simulink model "mrefrobotarm_modified_previous_y_previous_u_previous_ref_Thao"  (R2018b)
settings: Solver=FixedStepAuto  StartTime=0.0  StopTime=10  RelTol=1e-3  AbsTol=1e-6
undefined symbols (not defined in the file or in its folder): sfunxy2
libraries: neural x668, simulink x1
(part 16 of 21)

== system mrefrobotarm_modified_previous_y_previous_u_previous_ref_Thao/trimmed_2_report/Layer 2/Delays 1 ==
  "p{2}" : Inport  PortDimensions=50
      mask Display: e = 0.06;c1 = [120 230 180]/255;c2 = ([120 230 180]+0)/(256+128);c3 = ([120 230 180]+128)/(256+128);patch([0 1 1 0],[0 0 1 1],c1);patch([0 1 1 1-e 1-e 0+e],[0 0 1 1-e 0+e 0+e],c2);patch([0 0 1 1-e 0+e 0+e],[0 1 1 1-e 1-e 0+e],c3);plot([0 1 1 0 0],[0 0 1 1 0]);
  mux : Mux  Inputs=1
      mask Display: e = 0.06;c1 = [120 150 230]/255;c2 = ([120 150 230]+0)/383;c3 = ([120 150 230]+128)/383;patch([0 1 1 0],[0 0 1 1],c1);patch([0 1 1 1-e 1-e 0+e],[0 0 1 1-e 0+e 0+e],c2);patch([0 0 1 1-e 0+e 0+e],[0 1 1 1-e 1-e 0+e],c3);plot([0 1 1 0 0],[0 0 1 1 0]);disp('Mux')
  "pd{2,1}" : Outport
      mask Display: e = 0.06;c1 = [120 230 180]/255;c2 = ([120 230 180]+0)/(256+128);c3 = ([120 230 180]+128)/(256+128);patch([0 1 1 0],[0 0 1 1],c1);patch([0 1 1 1-e 1-e 0+e],[0 0 1 1-e 0+e 0+e],c2);patch([0 0 1 1-e 0+e 0+e],[0 1 1 1-e 1-e 0+e],c3);plot([0 1 1 0 0],[0 0 1 1 0]);
  wires:
  "p{2}"/1 -> mux/1
  mux/1 -> "pd{2,1}"/1

== system mrefrobotarm_modified_previous_y_previous_u_previous_ref_Thao/trimmed_2_report/Layer 2/LW{2,1} ==
  "ad{2,1}" : Inport  PortDimensions=50
      mask Display: e = 0.06;c1 = [120 230 180]/255;c2 = ([120 230 180]+0)/(256+128);c3 = ([120 230 180]+128)/(256+128);patch([0 1 1 0],[0 0 1 1],c1);patch([0 1 1 1-e 1-e 0+e],[0 0 1 1-e 0+e 0+e],c2);patch([0 0 1 1-e 0+e 0+e],[0 1 1 1-e 1-e 0+e],c3);plot([0 1 1 0 0],[0 0 1 1 0]);
  "IW{2,1}(1,:)'" : Constant  Value=[-0.534499281996474007172537312726490199565887451171875;0.050521392035346612825463807894266210496425628662109375;-0.1237457148938286011219389592952211387455463409423828125;0.27380803107087559045140778835047967731952667236328125;-0.158040380072445307835238281768397428095340728759765625;0.0117056595849677480547512686825939454138278961181640625;0.0221259878671266306537912527119260630570352077484130859375;-0.021458436433733317494354508880860521458089351654052734375;0.51989139454196420242482190587907098233699798583984375;0.227624128585074136932320243431604467332363128662109375;0.01291812527474923803783024567337633925490081310272216796875;0.394990958343573284050620486596017144620418548583984375;-0.31659097344442466148706216699793003499507904052734375;0.056111623746644932742011491200173622928559780120849609375;0.0645209389209373818108161913187359459698200225830078125;-0.026299150809179223931000279890213278122246265411376953125;-0.21062033219300591024847335575032047927379608154296875;0.4157878309067550848254768425249494612216949462890625;-0.1393911657788584890216299072562833316624164581298828125;0.007629605525119244335829904457568773068487644195556640625;-0.10964960705708633181831856973076355643570423126220703125;0.0231723744225558851705937257747791591100394725799560546875;-0.0049260595140393458046812469319775118492543697357177734375;-0.1840150338819656339328645344721735455095767974853515625;-0.102919672671898665416989615550846792757511138916015625;-0.00142893900606726360902332118030244600959122180938720703125;0.4164215191432472096266792505048215389251708984375;0.047497327884583662171991136347060091793537139892578125;-0.3258562173255992178155793226324021816253662109375;0.07218624218910708878471638172413804568350315093994140625;-0.000558610505585981249876414977961758268065750598907470703125;0.0227008210951530169097178912807066808454692363739013671875;0.004049470967297652025662646479986506165005266666412353515625;0.3794867924264113678844978494453243911266326904296875;-0.08706497710380935173279937089318991638720035552978515625;-0.299736725995607578010293536863173358142375946044921875;-0.046645176662323352412276022960213595069944858551025390625;0.2332394792535505689823338570931809954345226287841796875;0.0599754359488125776689315671319491229951381683349609375;0.158592158288105355978814259287901222705841064453125;0.061120750010903390769811949212453328073024749755859375;0.28961701664959627056106228337739594280719757080078125;0.057366268033513988233718094988944358192384243011474609375;0.05267609339257973977144189348109648562967777252197265625;0.0773590555953053982118916565013932995498180389404296875;-0.0394302645710693788760892175560002215206623077392578125;0.0381727970716883024948629099526442587375640869140625;-0.32777144511634259682608671937487088143825531005859375;0.329085099439463346637779750381014309823513031005859375;0.0716558723123885410455358169201645068824291229248046875]
      mask Display: e = 0.06;c1 = [120 150 230]/255;c2 = ([120 150 230]+0)/383;c3 = ([120 150 230]+128)/383;patch([0 1 1 0],[0 0 1 1],c1);patch([0 1 1 1-e 1-e 0+e],[0 0 1 1-e 0+e 0+e],c2);patch([0 0 1 1-e 0+e 0+e],[0 1 1 1-e 1-e 0+e],c3);plot([0 1 1 0 0],[0 0 1 1 0]);disp('weights');
  Mux : Mux  Inputs=1
      mask Display: e = 0.06;c1 = [120 150 230]/255;c2 = ([120 150 230]+0)/383;c3 = ([120 150 230]+128)/383;patch([0 1 1 0],[0 0 1 1],c1);patch([0 1 1 1-e 1-e 0+e],[0 0 1 1-e 0+e 0+e],c2);patch([0 0 1 1-e 0+e 0+e],[0 1 1 1-e 1-e 0+e],c3);plot([0 1 1 0 0],[0 0 1 1 0]);disp('Mux');
  dotprod1 : neural/Weight Functions/dotprod
  "lz{2,1}" : Outport
      mask Display: e = 0.06;c1 = [120 230 180]/255;c2 = ([120 230 180]+0)/(256+128);c3 = ([120 230 180]+128)/(256+128);patch([0 1 1 0],[0 0 1 1],c1);patch([0 1 1 1-e 1-e 0+e],[0 0 1 1-e 0+e 0+e],c2);patch([0 0 1 1-e 0+e 0+e],[0 1 1 1-e 1-e 0+e],c3);plot([0 1 1 0 0],[0 0 1 1 0]);
  wires:
  "IW{2,1}(1,:)'"/1 -> dotprod1/1
  "ad{2,1}"/1 -> dotprod1/2
  dotprod1/1 -> Mux/1
  Mux/1 -> "lz{2,1}"/1

== system mrefrobotarm_modified_previous_y_previous_u_previous_ref_Thao/trimmed_cex/Layer 1/Delays 1 ==
  "p{1}" : Inport  PortDimensions=10
      mask Display: e = 0.06;c1 = [120 230 180]/255;c2 = ([120 230 180]+0)/(256+128);c3 = ([120 230 180]+128)/(256+128);patch([0 1 1 0],[0 0 1 1],c1);patch([0 1 1 1-e 1-e 0+e],[0 0 1 1-e 0+e 0+e],c2);patch([0 0 1 1-e 0+e 0+e],[0 1 1 1-e 1-e 0+e],c3);plot([0 1 1 0 0],[0 0 1 1 0]);
  mux : Mux  Inputs=1
      mask Display: e = 0.06;c1 = [120 150 230]/255;c2 = ([120 150 230]+0)/383;c3 = ([120 150 230]+128)/383;patch([0 1 1 0],[0 0 1 1],c1);patch([0 1 1 1-e 1-e 0+e],[0 0 1 1-e 0+e 0+e],c2);patch([0 0 1 1-e 0+e 0+e],[0 1 1 1-e 1-e 0+e],c3);plot([0 1 1 0 0],[0 0 1 1 0]);disp('Mux')
  "pd{1,1}" : Outport
      mask Display: e = 0.06;c1 = [120 230 180]/255;c2 = ([120 230 180]+0)/(256+128);c3 = ([120 230 180]+128)/(256+128);patch([0 1 1 0],[0 0 1 1],c1);patch([0 1 1 1-e 1-e 0+e],[0 0 1 1-e 0+e 0+e],c2);patch([0 0 1 1-e 0+e 0+e],[0 1 1 1-e 1-e 0+e],c3);plot([0 1 1 0 0],[0 0 1 1 0]);
  wires:
  "p{1}"/1 -> mux/1
  mux/1 -> "pd{1,1}"/1

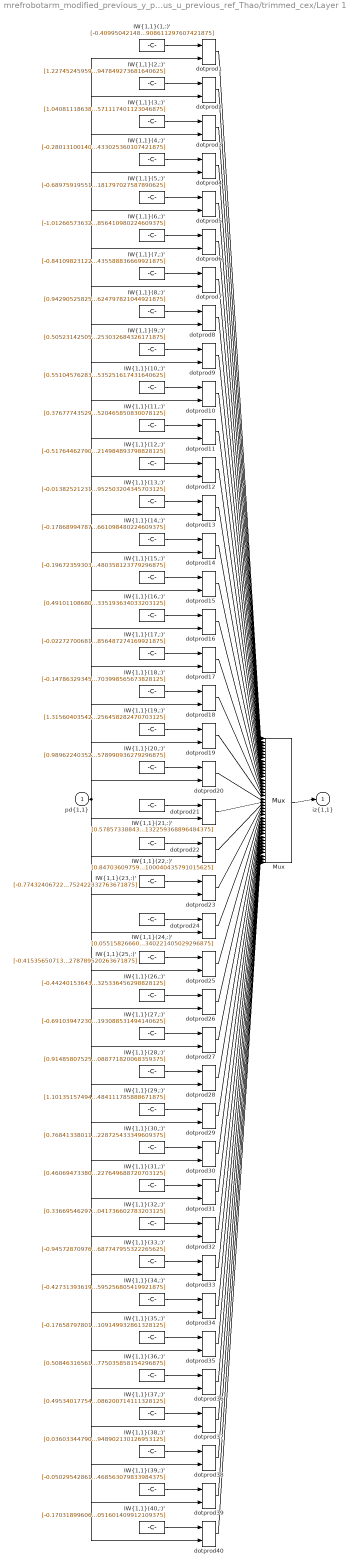
== system mrefrobotarm_modified_previous_y_previous_u_previous_ref_Thao/trimmed_cex/Layer 1/IW{1,1} ==
  "pd{1,1}" : Inport  PortDimensions=10
      mask Display: e = 0.06;c1 = [120 230 180]/255;c2 = ([120 230 180]+0)/(256+128);c3 = ([120 230 180]+128)/(256+128);patch([0 1 1 0],[0 0 1 1],c1);patch([0 1 1 1-e 1-e 0+e],[0 0 1 1-e 0+e 0+e],c2);patch([0 0 1 1-e 0+e 0+e],[0 1 1 1-e 1-e 0+e],c3);plot([0 1 1 0 0],[0 0 1 1 0]);
  "IW{1,1}(1,:)'" : Constant  Value=[-0.409950421486075355925748908703099004924297332763671875;-0.2664484226456824700335346278734505176544189453125;0.82215987443999594130872310415725223720073699951171875;-0.8070804278638721296346147937583737075328826904296875;-0.6354261914999630445066713946289382874965667724609375;0.93223383088760336523392879826133139431476593017578125;-0.478382274522026751384373710607178509235382080078125;-0.64553475014590000480296794194146059453487396240234375;0.60487535966275285392867999689769931137561798095703125;-0.154506010113978298203818440015311352908611297607421875]
      mask Display: e = 0.06;c1 = [120 150 230]/255;c2 = ([120 150 230]+0)/383;c3 = ([120 150 230]+128)/383;patch([0 1 1 0],[0 0 1 1],c1);patch([0 1 1 1-e 1-e 0+e],[0 0 1 1-e 0+e 0+e],c2);patch([0 0 1 1-e 0+e 0+e],[0 1 1 1-e 1-e 0+e],c3);plot([0 1 1 0 0],[0 0 1 1 0]);disp('Weights');
  "IW{1,1}(10,:)'" : Constant  Value=[0.55104576283990980289928529600729234516620635986328125;0.70635327144264181686850179175962693989276885986328125;1.0688781204485005016380227971239946782588958740234375;0.2351630117278747655884529876857413910329341888427734375;0.18201702354305349107477240977459587156772613525390625;-0.55143005136851630521022116226959042251110076904296875;-0.86246809425289316930474114997196011245250701904296875;-0.9777826678231626988946345591102726757526397705078125;0.74981547833765638255698604552890174090862274169921875;0.55583250060019795402155295960255898535251617431640625]
      mask Display: e = 0.06;c1 = [120 150 230]/255;c2 = ([120 150 230]+0)/383;c3 = ([120 150 230]+128)/383;patch([0 1 1 0],[0 0 1 1],c1);patch([0 1 1 1-e 1-e 0+e],[0 0 1 1-e 0+e 0+e],c2);patch([0 0 1 1-e 0+e 0+e],[0 1 1 1-e 1-e 0+e],c3);plot([0 1 1 0 0],[0 0 1 1 0]);disp('Weights');
  "IW{1,1}(11,:)'" : Constant  Value=[0.3767774352905917112366296350955963134765625;0.2009752253063678828493010541933472268283367156982421875;-0.89354895099178488493407712667249143123626708984375;0.6899875287137533508285969219286926090717315673828125;1.125933724805846747329951540450565516948699951171875;0.54802615696479095586113317040144465863704681396484375;0.38602265314686545760736180454841814935207366943359375;-0.31980146358828631658610675003728829324245452880859375;-1.0052964528057055648702089456492103636264801025390625;0.327354157170351378614014947743271477520465850830078125]
      mask Display: e = 0.06;c1 = [120 150 230]/255;c2 = ([120 150 230]+0)/383;c3 = ([120 150 230]+128)/383;patch([0 1 1 0],[0 0 1 1],c1);patch([0 1 1 1-e 1-e 0+e],[0 0 1 1-e 0+e 0+e],c2);patch([0 0 1 1-e 0+e 0+e],[0 1 1 1-e 1-e 0+e],c3);plot([0 1 1 0 0],[0 0 1 1 0]);disp('Weights');
  "IW{1,1}(12,:)'" : Constant  Value=[-0.5176446279089115254379294128739275038242340087890625;0.74329648028114936320065453401184640824794769287109375;0.56129611953699132254058667967910878360271453857421875;0.6656237941179730110974333001649938523769378662109375;0.17927298805446090224080535335815511643886566162109375;1.010790447986693152415682561695575714111328125;0.8347516775559349344604243015055544674396514892578125;-0.2256657861482148919041179624400683678686618804931640625;0.2438529279834821539285627522986033000051975250244140625;0.79710465235954064411316721816547214984893798828125]
      mask Display: e = 0.06;c1 = [120 150 230]/255;c2 = ([120 150 230]+0)/383;c3 = ([120 150 230]+128)/383;patch([0 1 1 0],[0 0 1 1],c1);patch([0 1 1 1-e 1-e 0+e],[0 0 1 1-e 0+e 0+e],c2);patch([0 0 1 1-e 0+e 0+e],[0 1 1 1-e 1-e 0+e],c3);plot([0 1 1 0 0],[0 0 1 1 0]);disp('Weights');
  "IW{1,1}(13,:)'" : Constant  Value=[-0.0138252123130195199440795050804808852262794971466064453125;0.7310768485028218410803901861072517931461334228515625;0.1793313597198371578400610815151594579219818115234375;0.03382004408312382082169023078677128069102764129638671875;-1.7686173826988913493352129080449230968952178955078125;-0.25051326753296521143710151591221801936626434326171875;1.213436044436186467265770261292345821857452392578125;0.26416181179519904187458223532303236424922943115234375;-0.2117864442757750598200772174095618538558483123779296875;-0.43316444584072766321725111993146128952503204345703125]
      mask Display: e = 0.06;c1 = [120 150 230]/255;c2 = ([120 150 230]+0)/383;c3 = ([120 150 230]+128)/383;patch([0 1 1 0],[0 0 1 1],c1);patch([0 1 1 1-e 1-e 0+e],[0 0 1 1-e 0+e 0+e],c2);patch([0 0 1 1-e 0+e 0+e],[0 1 1 1-e 1-e 0+e],c3);plot([0 1 1 0 0],[0 0 1 1 0]);disp('Weights');
  "IW{1,1}(14,:)'" : Constant  Value=[-0.178689947872833265751779663332854397594928741455078125;-0.6214830678008553821456416699220426380634307861328125;0.301565599171200349193355805255123414099216461181640625;0.282215738197436449841148942141444422304630279541015625;-1.235070373536440779815848145517520606517791748046875;0.0018266847157617609187507667911631870083510875701904296875;0.0304094742715033151958525792224463657476007938385009765625;0.9682731964107362809812684645294211804866790771484375;0.63588548799484378992730171376024372875690460205078125;0.79038843670227298954245043205446563661098480224609375]
      mask Display: e = 0.06;c1 = [120 150 230]/255;c2 = ([120 150 230]+0)/383;c3 = ([120 150 230]+128)/383;patch([0 1 1 0],[0 0 1 1],c1);patch([0 1 1 1-e 1-e 0+e],[0 0 1 1-e 0+e 0+e],c2);patch([0 0 1 1-e 0+e 0+e],[0 1 1 1-e 1-e 0+e],c3);plot([0 1 1 0 0],[0 0 1 1 0]);disp('Weights');
  "IW{1,1}(15,:)'" : Constant  Value=[-0.1967235930329597481946990455980994738638401031494140625;0.4999398005660731225674453526153229176998138427734375;0.89412234324233430537987032948876731097698211669921875;0.05945266912088405242275968021203880198299884796142578125;0.0474482273376281848964453047301503829658031463623046875;0.3036461092060902533518174095661379396915435791015625;-0.15896471182623905793462881774757988750934600830078125;-0.9253496196720145672287571869674138724803924560546875;0.918719060230821948920265640481375157833099365234375;-0.900185313959386501636572575080208480358123779296875]
      mask Display: e = 0.06;c1 = [120 150 230]/255;c2 = ([120 150 230]+0)/383;c3 = ([120 150 230]+128)/383;patch([0 1 1 0],[0 0 1 1],c1);patch([0 1 1 1-e 1-e 0+e],[0 0 1 1-e 0+e 0+e],c2);patch([0 0 1 1-e 0+e 0+e],[0 1 1 1-e 1-e 0+e],c3);plot([0 1 1 0 0],[0 0 1 1 0]);disp('Weights');
  "IW{1,1}(16,:)'" : Constant  Value=[0.491011086807734031811634167752345092594623565673828125;0.155186933005624305703662457744940184056758880615234375;-0.11711099155229769130937000909398193471133708953857421875;-0.66276689623297635467480404258822090923786163330078125;-0.5422964498312499159737853915430605411529541015625;0.304146121397555424525904754773364402353763580322265625;0.887358139122755407157683293917216360569000244140625;-0.99099461583372683293191585107706487178802490234375;0.3830059630076496635098237675265409052371978759765625;0.27587055069574983878766261113923974335193634033203125]
      mask Display: e = 0.06;c1 = [120 150 230]/255;c2 = ([120 150 230]+0)/383;c3 = ([120 150 230]+128)/383;patch([0 1 1 0],[0 0 1 1],c1);patch([0 1 1 1-e 1-e 0+e],[0 0 1 1-e 0+e 0+e],c2);patch([0 0 1 1-e 0+e 0+e],[0 1 1 1-e 1-e 0+e],c3);plot([0 1 1 0 0],[0 0 1 1 0]);disp('Weights');
  "IW{1,1}(17,:)'" : Constant  Value=[-0.0227270068157796149843630217901591095142066478729248046875;-0.0033446203266591680025587862701286212541162967681884765625;0.555597040712585421573521671234630048274993896484375;0.4055619247689070672180378096527419984340667724609375;-0.69873436239766750777135939642903394997119903564453125;-0.69174437201428318200413514205138199031352996826171875;-0.14958891890921821588023021831759251654148101806640625;1.146594252841719008273457802715711295604705810546875;1.0912485097967479230618437213706783950328826904296875;0.69285833323481404999455435245181433856487274169921875]
      mask Display: e = 0.06;c1 = [120 150 230]/255;c2 = ([120 150 230]+0)/383;c3 = ([120 150 230]+128)/383;patch([0 1 1 0],[0 0 1 1],c1);patch([0 1 1 1-e 1-e 0+e],[0 0 1 1-e 0+e 0+e],c2);patch([0 0 1 1-e 0+e 0+e],[0 1 1 1-e 1-e 0+e],c3);plot([0 1 1 0 0],[0 0 1 1 0]);disp('Weights');
  "IW{1,1}(18,:)'" : Constant  Value=[-0.1478632934526930842178416014576214365661144256591796875;-0.3452155889878729677633373285061679780483245849609375;-0.0966016042904927763057543188551790080964565277099609375;-0.56056969383534227535648142293212004005908966064453125;-1.499417823985652820084624181617982685565948486328125;0.89052501293365116108446954967803321778774261474609375;-0.5465292024094947631596141945919953286647796630859375;0.54948094360087551546456552387098781764507293701171875;0.08803384133689766410935106932811322622001171112060546875;0.561317847656468860151335320551879703998565673828125]
      mask Display: e = 0.06;c1 = [120 150 230]/255;c2 = ([120 150 230]+0)/383;c3 = ([120 150 230]+128)/383;patch([0 1 1 0],[0 0 1 1],c1);patch([0 1 1 1-e 1-e 0+e],[0 0 1 1-e 0+e 0+e],c2);patch([0 0 1 1-e 0+e 0+e],[0 1 1 1-e 1-e 0+e],c3);plot([0 1 1 0 0],[0 0 1 1 0]);disp('Weights');
  "IW{1,1}(19,:)'" : Constant  Value=[1.31560403542571524582172060036100447177886962890625;0.8777692427769456795516589409089647233486175537109375;-0.205947039131328335503923199212295003235340118408203125;0.498609152543595890438865581018035300076007843017578125;-0.01839913800753746608851457722266786731779575347900390625;-0.498700799665831306928254207377904094755649566650390625;-0.42702038547360976483702188488678075373172760009765625;0.98979145575477545104803311915020458400249481201171875;0.096199212682389123596493618606473319232463836669921875;-0.2748632724632014134868995824945159256458282470703125]
      mask Display: e = 0.06;c1 = [120 150 230]/255;c2 = ([120 150 230]+0)/383;c3 = ([120 150 230]+128)/383;patch([0 1 1 0],[0 0 1 1],c1);patch([0 1 1 1-e 1-e 0+e],[0 0 1 1-e 0+e 0+e],c2);patch([0 0 1 1-e 0+e 0+e],[0 1 1 1-e 1-e 0+e],c3);plot([0 1 1 0 0],[0 0 1 1 0]);disp('Weights');
  "IW{1,1}(2,:)'" : Constant  Value=[1.2274524595998828058185381451039575040340423583984375;-0.1858982387281616077689960775387589819729328155517578125;0.028275394747831437969320944603168754838407039642333984375;0.0847112914180939979846840515165240503847599029541015625;-1.1893226383913002575098971647094003856182098388671875;-0.06498424728492711854865859777419245801866054534912109375;1.1521911516761191851543344455421902239322662353515625;-0.285463137559759216888011224000365473330020904541015625;-1.181173392303688896021185428253374993801116943359375;-0.6258040532702013880594904549070633947849273681640625]
      mask Display: e = 0.06;c1 = [120 150 230]/255;c2 = ([120 150 230]+0)/383;c3 = ([120 150 230]+128)/383;patch([0 1 1 0],[0 0 1 1],c1);patch([0 1 1 1-e 1-e 0+e],[0 0 1 1-e 0+e 0+e],c2);patch([0 0 1 1-e 0+e 0+e],[0 1 1 1-e 1-e 0+e],c3);plot([0 1 1 0 0],[0 0 1 1 0]);disp('Weights');
  "IW{1,1}(20,:)'" : Constant  Value=[0.9896224035276339758837593763018958270549774169921875;-0.44305668527520125632435110674123279750347137451171875;0.70981606561427990076396099539124406874179840087890625;-1.1297168139596982516792422757134772837162017822265625;0.848697028814358045423205112456344068050384521484375;0.4557425970205557508307947500725276768207550048828125;-0.39557951689199721823086974836769513785839080810546875;-0.00146782704480703796168228336682659573853015899658203125;0.2214522806691265888190400801249779760837554931640625;-0.132984556624309024908114906793343834578990936279296875]
      mask Display: e = 0.06;c1 = [120 150 230]/255;c2 = ([120 150 230]+0)/383;c3 = ([120 150 230]+128)/383;patch([0 1 1 0],[0 0 1 1],c1);patch([0 1 1 1-e 1-e 0+e],[0 0 1 1-e 0+e 0+e],c2);patch([0 0 1 1-e 0+e 0+e],[0 1 1 1-e 1-e 0+e],c3);plot([0 1 1 0 0],[0 0 1 1 0]);disp('Weights');
  "IW{1,1}(21,:)'" : Constant  Value=[0.57857338843473637979286650079302489757537841796875;0.55341504998858115360604870147653855383396148681640625;-0.64653962666199527031807292587473057210445404052734375;-0.5862476181018936305378019824274815618991851806640625;-0.35438450623822148610742033270071260631084442138671875;0.510302004487602101079346539336256682872772216796875;-0.9929389094367564450038798895548097789287567138671875;-0.74814260248213215742651982509414665400981903076171875;-0.90267234096774806584306816148455254733562469482421875;0.423604583182045801859061384675442241132259368896484375]
      mask Display: e = 0.06;c1 = [120 150 230]/255;c2 = ([120 150 230]+0)/383;c3 = ([120 150 230]+128)/383;patch([0 1 1 0],[0 0 1 1],c1);patch([0 1 1 1-e 1-e 0+e],[0 0 1 1-e 0+e 0+e],c2);patch([0 0 1 1-e 0+e 0+e],[0 1 1 1-e 1-e 0+e],c3);plot([0 1 1 0 0],[0 0 1 1 0]);disp('Weights');
  "IW{1,1}(22,:)'" : Constant  Value=[0.84703609759596532047254413555492646992206573486328125;-0.7880910829087459656960845677531324326992034912109375;-0.6116141806369055355929731376818381249904632568359375;-0.72231053399220801480851150699891149997711181640625;-0.6838583880533806169665922425338067114353179931640625;0.45809248458162443728980406376649625599384307861328125;-0.46923654407256443210627594453399069607257843017578125;-0.489852123921882542934014281854615546762943267822265625;-0.84453888161475798579402862742426805198192596435546875;0.2119728726749436076293164887829334475100040435791015625]
      mask Display: e = 0.06;c1 = [120 150 230]/255;c2 = ([120 150 230]+0)/383;c3 = ([120 150 230]+128)/383;patch([0 1 1 0],[0 0 1 1],c1);patch([0 1 1 1-e 1-e 0+e],[0 0 1 1-e 0+e 0+e],c2);patch([0 0 1 1-e 0+e 0+e],[0 1 1 1-e 1-e 0+e],c3);plot([0 1 1 0 0],[0 0 1 1 0]);disp('Weights');
  "IW{1,1}(23,:)'" : Constant  Value=[-0.77432406722360103135116560224560089409351348876953125;0.2209649232498732962515219924171105958521366119384765625;0.46444341998348026567811075437930412590503692626953125;-0.6595292492139612772206191948498599231243133544921875;0.134455139336463080912409395750728435814380645751953125;-1.10985874298612419153187147458083927631378173828125;-1.12233395519971512754864306771196424961090087890625;1.1289026833873487820625314270728267729282379150390625;0.49296594290608830579714094710652716457843780517578125;-0.1470205149079321926830488109771977178752422332763671875]
      mask Display: e = 0.06;c1 = [120 150 230]/255;c2 = ([120 150 230]+0)/383;c3 = ([120 150 230]+128)/383;patch([0 1 1 0],[0 0 1 1],c1);patch([0 1 1 1-e 1-e 0+e],[0 0 1 1-e 0+e 0+e],c2);patch([0 0 1 1-e 0+e 0+e],[0 1 1 1-e 1-e 0+e],c3);plot([0 1 1 0 0],[0 0 1 1 0]);disp('Weights');
  "IW{1,1}(24,:)'" : Constant  Value=[0.0551582666045678238209148958048899658024311065673828125;-0.2255705806114211287027870866950252093374729156494140625;-0.1126119364538074318904392612239462323486804962158203125;-0.7413220356632257423967757858918048441410064697265625;0.54959437813839329134424360745470039546489715576171875;0.94089820560549319861110006968374364078044891357421875;-0.2087613420724725721289161128879641182720661163330078125;-0.0106507648017074955937300018149471725337207317352294921875;1.180621398067102756357371617923490703105926513671875;-0.9673907138311139686237538626301102340221405029296875]
      mask Display: e = 0.06;c1 = [120 150 230]/255;c2 = ([120 150 230]+0)/383;c3 = ([120 150 230]+128)/383;patch([0 1 1 0],[0 0 1 1],c1);patch([0 1 1 1-e 1-e 0+e],[0 0 1 1-e 0+e 0+e],c2);patch([0 0 1 1-e 0+e 0+e],[0 1 1 1-e 1-e 0+e],c3);plot([0 1 1 0 0],[0 0 1 1 0]);disp('Weights');
  "IW{1,1}(25,:)'" : Constant  Value=[-0.415356507133745889159825992464902810752391815185546875;0.86324940583818221551126725898939184844493865966796875;0.99650446455441699100674668443389236927032470703125;1.240869987062364732111063858610577881336212158203125;-0.2453879737701236962710282796251703985035419464111328125;0.09212383002728556646854229938981006853282451629638671875;-0.6468176112671486510663498847861774265766143798828125;-0.34821678674260481134439260131330229341983795166015625;-0.641556475722417030027600048924796283245086669921875;0.284721166353878174515301680003176443278789520263671875]
      mask Display: e = 0.06;c1 = [120 150 230]/255;c2 = ([120 150 230]+0)/383;c3 = ([120 150 230]+128)/383;patch([0 1 1 0],[0 0 1 1],c1);patch([0 1 1 1-e 1-e 0+e],[0 0 1 1-e 0+e 0+e],c2);patch([0 0 1 1-e 0+e 0+e],[0 1 1 1-e 1-e 0+e],c3);plot([0 1 1 0 0],[0 0 1 1 0]);disp('Weights');
  "IW{1,1}(26,:)'" : Constant  Value=[-0.44240153643942903283203804676304571330547332763671875;0.59430493538216089266512653921381570398807525634765625;0.5394873214608788547508311239653266966342926025390625;0.954342632885547548227123115793801844120025634765625;1.2058311250139173154138916288502514362335205078125;-0.0323482288472860257666496863748761825263500213623046875;-0.42951089724954016890734465050627477467060089111328125;-0.6539844271651749085805249706027098000049591064453125;-0.92613626911378787998074813003768213093280792236328125;0.51958222819110588819313534258981235325336456298828125]
      mask Display: e = 0.06;c1 = [120 150 230]/255;c2 = ([120 150 230]+0)/383;c3 = ([120 150 230]+128)/383;patch([0 1 1 0],[0 0 1 1],c1);patch([0 1 1 1-e 1-e 0+e],[0 0 1 1-e 0+e 0+e],c2);patch([0 0 1 1-e 0+e 0+e],[0 1 1 1-e 1-e 0+e],c3);plot([0 1 1 0 0],[0 0 1 1 0]);disp('Weights');
  "IW{1,1}(27,:)'" : Constant  Value=[-0.6910394723013333351246956226532347500324249267578125;0.1300887580630211426413467279417091049253940582275390625;0.59345223422897108722651182688423432409763336181640625;0.51550685897836279192318897912628017365932464599609375;0.93137492332801341543557782642892561852931976318359375;-0.9162873587680151477030676687718369066715240478515625;-0.17297120305768209913566124669159762561321258544921875;-0.8593544727265882698929999605752527713775634765625;0.1586520633134883284665050950934528373181819915771484375;-0.55374611924893957226601060028770007193088531494140625]
      mask Display: e = 0.06;c1 = [120 150 230]/255;c2 = ([120 150 230]+0)/383;c3 = ([120 150 230]+128)/383;patch([0 1 1 0],[0 0 1 1],c1);patch([0 1 1 1-e 1-e 0+e],[0 0 1 1-e 0+e 0+e],c2);patch([0 0 1 1-e 0+e 0+e],[0 1 1 1-e 1-e 0+e],c3);plot([0 1 1 0 0],[0 0 1 1 0]);disp('Weights');
  "IW{1,1}(28,:)'" : Constant  Value=[0.9148580752542054828069240102195180952548980712890625;0.47950481890905793935786505244323052465915679931640625;-0.2490172912492536472228721322608180344104766845703125;-0.4966378241611513200126637457287870347499847412109375;-0.9368352984117274129260977133526466786861419677734375;-0.0244576534631735405256325321943222661502659320831298828125;0.6703792015266636372672337529365904629230499267578125;0.264773753200862105305901650353916920721530914306640625;-0.72082279686418360142852179706096649169921875;-0.8897551832598364907056520678452216088771820068359375]
      mask Display: e = 0.06;c1 = [120 150 230]/255;c2 = ([120 150 230]+0)/383;c3 = ([120 150 230]+128)/383;patch([0 1 1 0],[0 0 1 1],c1);patch([0 1 1 1-e 1-e 0+e],[0 0 1 1-e 0+e 0+e],c2);patch([0 0 1 1-e 0+e 0+e],[0 1 1 1-e 1-e 0+e],c3);plot([0 1 1 0 0],[0 0 1 1 0]);disp('Weights');
  "IW{1,1}(29,:)'" : Constant  Value=[1.1013515749485349726199956421623937785625457763671875;0.06693104392684272319069549439518596045672893524169921875;-0.5772231018648612543842091326951049268245697021484375;-0.70668665976109357185208637019968591630458831787109375;0.054245178681219897998122547733146348036825656890869140625;1.17995645249989156155834280070848762989044189453125;-0.40163239637189784847493001507245935499668121337890625;0.51426896753677586726638537584221921861171722412109375;-0.368155350470345699154250951323774643242359161376953125;-0.51608120747988805998573980104993097484111785888671875]
      mask Display: e = 0.06;c1 = [120 150 230]/255;c2 = ([120 150 230]+0)/383;c3 = ([120 150 230]+128)/383;patch([0 1 1 0],[0 0 1 1],c1);patch([0 1 1 1-e 1-e 0+e],[0 0 1 1-e 0+e 0+e],c2);patch([0 0 1 1-e 0+e 0+e],[0 1 1 1-e 1-e 0+e],c3);plot([0 1 1 0 0],[0 0 1 1 0]);disp('Weights');
  "IW{1,1}(3,:)'" : Constant  Value=[1.0408111863854216938563013172824867069721221923828125;-0.283621341010957095374322989300708286464214324951171875;0.58923441896435646558671805905760265886783599853515625;0.5656313215120396531432334086275659501552581787109375;0.270988613432589231511116167894215323030948638916015625;-0.842745168324875226772974201594479382038116455078125;-0.039030976236690016756281096377279027365148067474365234375;-0.74611980012757495028807852577301673591136932373046875;-0.1793432692938618788769389311710256151854991912841796875;-0.84794562302679021836837591763469390571117401123046875]
      mask Display: e = 0.06;c1 = [120 150 230]/255;c2 = ([120 150 230]+0)/383;c3 = ([120 150 230]+128)/383;patch([0 1 1 0],[0 0 1 1],c1);patch([0 1 1 1-e 1-e 0+e],[0 0 1 1-e 0+e 0+e],c2);patch([0 0 1 1-e 0+e 0+e],[0 1 1 1-e 1-e 0+e],c3);plot([0 1 1 0 0],[0 0 1 1 0]);disp('Weights');
  "IW{1,1}(30,:)'" : Constant  Value=[0.76841338011237081406790139226359315216541290283203125;-0.26203413140045783702447579344152472913265228271484375;-0.11137080922380983294406320283087552525103092193603515625;0.86629343686568460736197039295802824199199676513671875;-0.453692803926102505851503110534395091235637664794921875;-0.0169754124456641709850490684630130999721586704254150390625;-0.84262937452250918912710631047957576811313629150390625;0.053251670861151449709591787495810422115027904510498046875;0.59034214461825762487734436945174820721149444580078125;0.9439979223442553912803987259394489228725433349609375]
      mask Display: e = 0.06;c1 = [120 150 230]/255;c2 = ([120 150 230]+0)/383;c3 = ([120 150 230]+128)/383;patch([0 1 1 0],[0 0 1 1],c1);patch([0 1 1 1-e 1-e 0+e],[0 0 1 1-e 0+e 0+e],c2);patch([0 0 1 1-e 0+e 0+e],[0 1 1 1-e 1-e 0+e],c3);plot([0 1 1 0 0],[0 0 1 1 0]);disp('Weights');
  "IW{1,1}(31,:)'" : Constant  Value=[0.460694733802664180277730565649108029901981353759765625;-0.53047192158973943687527707879780791699886322021484375;0.8159974818512891747701587519259192049503326416015625;0.718033038612972074332674310426227748394012451171875;0.913543940794618425371709236060269176959991455078125;0.054591792642314486416754704123377450741827487945556640625;0.7305929664212273966228394783684052526950836181640625;0.544299193225226130010696579120121896266937255859375;-0.2431177138067444343239031923076254315674304962158203125;-0.98559135751877502418238918835413642227649688720703125]
      mask Display: e = 0.06;c1 = [120 150 230]/255;c2 = ([120 150 230]+0)/383;c3 = ([120 150 230]+128)/383;patch([0 1 1 0],[0 0 1 1],c1);patch([0 1 1 1-e 1-e 0+e],[0 0 1 1-e 0+e 0+e],c2);patch([0 0 1 1-e 0+e 0+e],[0 1 1 1-e 1-e 0+e],c3);plot([0 1 1 0 0],[0 0 1 1 0]);disp('Weights');
  "IW{1,1}(32,:)'" : Constant  Value=[0.33669546297750929664260866047698073089122772216796875;1.1460294404612714203040013671852648258209228515625;-0.37550081912030019992698726127855479717254638671875;-0.384303972314102126883739174445508979260921478271484375;-0.360178495564217493463132768738432787358760833740234375;-0.60626011569394144817835012872819788753986358642578125;0.94114892334687028085937754440237767994403839111328125;0.7851101225738339461912573824520222842693328857421875;-0.54980880337690163361941131370258517563343048095703125;-0.3363615159827741951659163532895036041736602783203125]
      mask Display: e = 0.06;c1 = [120 150 230]/255;c2 = ([120 150 230]+0)/383;c3 = ([120 150 230]+128)/383;patch([0 1 1 0],[0 0 1 1],c1);patch([0 1 1 1-e 1-e 0+e],[0 0 1 1-e 0+e 0+e],c2);patch([0 0 1 1-e 0+e 0+e],[0 1 1 1-e 1-e 0+e],c3);plot([0 1 1 0 0],[0 0 1 1 0]);disp('Weights');
  "IW{1,1}(33,:)'" : Constant  Value=[-0.94572870976638390150270652156905271112918853759765625;-0.37474077493031876517903810963616706430912017822265625;-0.793913486234307352873429408646188676357269287109375;0.407177454893028534232968240758054889738559722900390625;0.408545047184475096369027369291870854794979095458984375;0.03994335791944710056800005304467049427330493927001953125;-0.8160403944444485357934127023327164351940155029296875;0.70046992525510898275342697161249816417694091796875;1.008882449885082355223175909486599266529083251953125;0.445674875484491028743150309310294687747955322265625]
      mask Display: e = 0.06;c1 = [120 150 230]/255;c2 = ([120 150 230]+0)/383;c3 = ([120 150 230]+128)/383;patch([0 1 1 0],[0 0 1 1],c1);patch([0 1 1 1-e 1-e 0+e],[0 0 1 1-e 0+e 0+e],c2);patch([0 0 1 1-e 0+e 0+e],[0 1 1 1-e 1-e 0+e],c3);plot([0 1 1 0 0],[0 0 1 1 0]);disp('Weights');
  "IW{1,1}(34,:)'" : Constant  Value=[-0.427313936195357790825966048942063935101032257080078125;0.222604386044569391156500159922870807349681854248046875;0.426481643660006515261784443282522261142730712890625;0.262747262183711749461423323737108148634433746337890625;1.024865343077669965765608139918185770511627197265625;0.437582278743387564912126208582776598632335662841796875;-0.12946691285127875925553553315694443881511688232421875;-1.051186123548690343199041308253072202205657958984375;0.59015069079801552032193967534112744033336639404296875;0.855828124119376365541711493278853595256805419921875]
      mask Display: e = 0.06;c1 = [120 150 230]/255;c2 = ([120 150 230]+0)/383;c3 = ([120 150 230]+128)/383;patch([0 1 1 0],[0 0 1 1],c1);patch([0 1 1 1-e 1-e 0+e],[0 0 1 1-e 0+e 0+e],c2);patch([0 0 1 1-e 0+e 0+e],[0 1 1 1-e 1-e 0+e],c3);plot([0 1 1 0 0],[0 0 1 1 0]);disp('Weights');
  "IW{1,1}(35,:)'" : Constant  Value=[-0.1765879780170026835950380927897640503942966461181640625;-0.5430825737402937836151295414310880005359649658203125;-0.71846810556134210745682366905384697020053863525390625;-0.62756883559493503721427032360224984586238861083984375;0.5271343845312994602636536001227796077728271484375;-0.92276224680604845840292682623839937150478363037109375;0.351792434375731044582380491192452609539031982421875;-0.76035270864267279211645700343069620430469512939453125;-0.5705602252666588380947132463916204869747161865234375;0.9782158893654611109269580992986448109149932861328125]
      mask Display: e = 0.06;c1 = [120 150 230]/255;c2 = ([120 150 230]+0)/383;c3 = ([120 150 230]+128)/383;patch([0 1 1 0],[0 0 1 1],c1);patch([0 1 1 1-e 1-e 0+e],[0 0 1 1-e 0+e 0+e],c2);patch([0 0 1 1-e 0+e 0+e],[0 1 1 1-e 1-e 0+e],c3);plot([0 1 1 0 0],[0 0 1 1 0]);disp('Weights');
  "IW{1,1}(36,:)'" : Constant  Value=[0.50846316561046311921501228425768204033374786376953125;-0.422411567478501559502745976715232245624065399169921875;-0.72055423055618472716332689742557704448699951171875;-0.837527041021212337312817908241413533687591552734375;-0.355438023646912404363007453866885043680667877197265625;-0.66517914368360642196620347021962516009807586669921875;-0.022562397986342776212698169047143892385065555572509765625;1.2141698888595573446735897960024885833263397216796875;-0.331376781169265777204913092646165750920772552490234375;-0.24466342991752643154512725232052616775035858154296875]
      mask Display: e = 0.06;c1 = [120 150 230]/255;c2 = ([120 150 230]+0)/383;c3 = ([120 150 230]+128)/383;patch([0 1 1 0],[0 0 1 1],c1);patch([0 1 1 1-e 1-e 0+e],[0 0 1 1-e 0+e 0+e],c2);patch([0 0 1 1-e 0+e 0+e],[0 1 1 1-e 1-e 0+e],c3);plot([0 1 1 0 0],[0 0 1 1 0]);disp('Weights');
  "IW{1,1}(37,:)'" : Constant  Value=[0.4953401775482857427590488441637717187404632568359375;-0.12108570130121835972669686043445835821330547332763671875;-0.1150513794768294462134150535348453558981418609619140625;0.9093488134476099826741801734897308051586151123046875;1.002065245884896871331193324294872581958770751953125;-0.272901586619709035641534455862711183726787567138671875;0.42695777633637554959733506620978005230426788330078125;-0.0925650898312258829658816239316365681588649749755859375;0.99915713808778428006718286269460804760456085205078125;0.842277767911099761732884871889837086200714111328125]
      mask Display: e = 0.06;c1 = [120 150 230]/255;c2 = ([120 150 230]+0)/383;c3 = ([120 150 230]+128)/383;patch([0 1 1 0],[0 0 1 1],c1);patch([0 1 1 1-e 1-e 0+e],[0 0 1 1-e 0+e 0+e],c2);patch([0 0 1 1-e 0+e 0+e],[0 1 1 1-e 1-e 0+e],c3);plot([0 1 1 0 0],[0 0 1 1 0]);disp('Weights');
  "IW{1,1}(38,:)'" : Constant  Value=[0.036033447900100268324052876778296194970607757568359375;-0.476183052767934988924736217086319811642169952392578125;-0.89931841364787523662727153350715525448322296142578125;-0.48811719670724962316654682581429369747638702392578125;0.444967708782716797610845560484449379146099090576171875;-0.92873960236668384737868109368719160556793212890625;-0.49632231482133926103728072121157310903072357177734375;0.5689638925643445421798105599009431898593902587890625;-0.78278552146573432413134696616907604038715362548828125;0.65497142396882968018445581037667579948902130126953125]
      mask Display: e = 0.06;c1 = [120 150 230]/255;c2 = ([120 150 230]+0)/383;c3 = ([120 150 230]+128)/383;patch([0 1 1 0],[0 0 1 1],c1);patch([0 1 1 1-e 1-e 0+e],[0 0 1 1-e 0+e 0+e],c2);patch([0 0 1 1-e 0+e 0+e],[0 1 1 1-e 1-e 0+e],c3);plot([0 1 1 0 0],[0 0 1 1 0]);disp('Weights');
  "IW{1,1}(39,:)'" : Constant  Value=[-0.0502954286197731248453379748752922751009464263916015625;-0.38959190228632645247586197001510299742221832275390625;-0.5794681673882042804990533113596029579639434814453125;-0.53802406214401055084550762330763973295688629150390625;1.7405216353267454199027497452334500849246978759765625;-1.0860280042544154799344369166647084057331085205078125;0.579337321970657459502263009198941290378570556640625;-0.0990206845459063733638771509504294954240322113037109375;-0.85065302613058701997061916699749417603015899658203125;-0.19206439842164202413954399162321351468563079833984375]
      mask Display: e = 0.06;c1 = [120 150 230]/255;c2 = ([120 150 230]+0)/383;c3 = ([120 150 230]+128)/383;patch([0 1 1 0],[0 0 1 1],c1);patch([0 1 1 1-e 1-e 0+e],[0 0 1 1-e 0+e 0+e],c2);patch([0 0 1 1-e 0+e 0+e],[0 1 1 1-e 1-e 0+e],c3);plot([0 1 1 0 0],[0 0 1 1 0]);disp('Weights');
  "IW{1,1}(4,:)'" : Constant  Value=[-0.2801310014058235875467062214738689363002777099609375;0.58441619993924420750630588372587226331233978271484375;-0.51587612785775605050986314381589181721210479736328125;0.28694938887101972824211770785041153430938720703125;-0.822295482884032313819488990702666342258453369140625;-0.93642181590818085457073038924136199057102203369140625;0.418965295195909914749421432134113274514675140380859375;-0.032808909180273980454867199796353816054761409759521484375;0.89790162745206936190101032480015419423580169677734375;-0.18399102067120132186772707427735440433025360107421875]
      mask Display: e = 0.06;c1 = [120 150 230]/255;c2 = ([120 150 230]+0)/383;c3 = ([120 150 230]+128)/383;patch([0 1 1 0],[0 0 1 1],c1);patch([0 1 1 1-e 1-e 0+e],[0 0 1 1-e 0+e 0+e],c2);patch([0 0 1 1-e 0+e 0+e],[0 1 1 1-e 1-e 0+e],c3);plot([0 1 1 0 0],[0 0 1 1 0]);disp('Weights');
  "IW{1,1}(40,:)'" : Constant  Value=[-0.17031899606498601684734239825047552585601806640625;-0.310331540268166838902885729112313129007816314697265625;-0.01007024130386899481159890257231381838209927082061767578125;-0.87241447254082571394206979675800539553165435791015625;-1.3523782329598434959194719340302981436252593994140625;0.81972917451892979290306584516656585037708282470703125;-0.37890865875833001918948639286099933087825775146484375;-0.5104193559530136869994976223097182810306549072265625;0.443385110247164260233176946712774224579334259033203125;0.790185975905122628404342322028242051601409912109375]
      mask Display: e = 0.06;c1 = [120 150 230]/255;c2 = ([120 150 230]+0)/383;c3 = ([120 150 230]+128)/383;patch([0 1 1 0],[0 0 1 1],c1);patch([0 1 1 1-e 1-e 0+e],[0 0 1 1-e 0+e 0+e],c2);patch([0 0 1 1-e 0+e 0+e],[0 1 1 1-e 1-e 0+e],c3);plot([0 1 1 0 0],[0 0 1 1 0]);disp('Weights');
  "IW{1,1}(5,:)'" : Constant  Value=[-0.6897591955173998368167076478130184113979339599609375;0.6475739711405805731914142597815953195095062255859375;0.67292405621340856125556229017092846333980560302734375;-0.691410547742746128818680517724715173244476318359375;0.28088128059196082464410437751212157309055328369140625;-0.911573539108160080246534562320448458194732666015625;0.097098884868539681036736510577611625194549560546875;0.4091046709434487116396894634817726910114288330078125;0.54382339414100033803123324105399660766124725341796875;-0.63886724157221730369116130532347597181797027587890625]
      mask Display: e = 0.06;c1 = [120 150 230]/255;c2 = ([120 150 230]+0)/383;c3 = ([120 150 230]+128)/383;patch([0 1 1 0],[0 0 1 1],c1);patch([0 1 1 1-e 1-e 0+e],[0 0 1 1-e 0+e 0+e],c2);patch([0 0 1 1-e 0+e 0+e],[0 1 1 1-e 1-e 0+e],c3);plot([0 1 1 0 0],[0 0 1 1 0]);disp('Weights');
  "IW{1,1}(6,:)'" : Constant  Value=[-1.0126657363224402796930689873988740146160125732421875;0.450539092153614484370649506672634743154048919677734375;0.7922505445187797423756137504824437201023101806640625;0.61488298518615958077049299390637315809726715087890625;-0.56197764229621338660791707297903485596179962158203125;-0.06065491824535902687376420772125129587948322296142578125;0.83519747003309319222097428792039863765239715576171875;0.017225910397417755481885848212186829186975955963134765625;0.9511415910036102872027186094783246517181396484375;-0.56885108819651042377785188364214263856410980224609375]
      mask Display: e = 0.06;c1 = [120 150 230]/255;c2 = ([120 150 230]+0)/383;c3 = ([120 150 230]+128)/383;patch([0 1 1 0],[0 0 1 1],c1);patch([0 1 1 1-e 1-e 0+e],[0 0 1 1-e 0+e 0+e],c2);patch([0 0 1 1-e 0+e 0+e],[0 1 1 1-e 1-e 0+e],c3);plot([0 1 1 0 0],[0 0 1 1 0]);disp('Weights');
  "IW{1,1}(7,:)'" : Constant  Value=[-0.841098231229458814794952559168450534343719482421875;-0.204086836371817736957012812126777134835720062255859375;0.30525589456136881238990099518559873104095458984375;0.381161175733835289047846117682638578116893768310546875;-0.55600815285631977058500297061982564628124237060546875;-0.313544891190427055249756449484266340732574462890625;1.0570639441288818272113303464720956981182098388671875;-0.86615393045327682131073743221350014209747314453125;-0.6691997243019811580921896165818907320499420166015625;-0.000343398163943648446032319565546231387997977435588836669921875]
      mask Display: e = 0.06;c1 = [120 150 230]/255;c2 = ([120 150 230]+0)/383;c3 = ([120 150 230]+128)/383;patch([0 1 1 0],[0 0 1 1],c1);patch([0 1 1 1-e 1-e 0+e],[0 0 1 1-e 0+e 0+e],c2);patch([0 0 1 1-e 0+e 0+e],[0 1 1 1-e 1-e 0+e],c3);plot([0 1 1 0 0],[0 0 1 1 0]);disp('Weights');
  "IW{1,1}(8,:)'" : Constant  Value=[0.94290525825133852944048840072355233132839202880859375;-0.0282436591152728268261373756331522599793970584869384765625;-0.33209169421805240229872424606583081185817718505859375;0.9974843995064048840504256077110767364501953125;0.6625406877042145925571503539686091244220733642578125;-0.8553382057199530041913249078788794577121734619140625;-0.5484685443330208354240085100173018872737884521484375;-0.67658319089995855311059358427883125841617584228515625;-0.394762151505675007445717028531362302601337432861328125;0.45336774475889007884887860200251452624797821044921875]
      mask Display: e = 0.06;c1 = [120 150 230]/255;c2 = ([120 150 230]+0)/383;c3 = ([120 150 230]+128)/383;patch([0 1 1 0],[0 0 1 1],c1);patch([0 1 1 1-e 1-e 0+e],[0 0 1 1-e 0+e 0+e],c2);patch([0 0 1 1-e 0+e 0+e],[0 1 1 1-e 1-e 0+e],c3);plot([0 1 1 0 0],[0 0 1 1 0]);disp('Weights');
  "IW{1,1}(9,:)'" : Constant  Value=[0.50523142505917373323853780675563029944896697998046875;0.0883511673375003692143536682124249637126922607421875;0.8811374363621455874096000115969218313694000244140625;-1.120039010118599520637872046791017055511474609375;-0.259255439009866084365540928047266788780689239501953125;0.76066577143904334779023201917880214750766754150390625;0.1438890698550478186579226758112781681120395660400390625;0.43908453789031220981797787317191250622272491455078125;0.8333800756497049544435640200390480458736419677734375;-0.09288028783054440296051978975810925476253032684326171875]
      mask Display: e = 0.06;c1 = [120 150 230]/255;c2 = ([120 150 230]+0)/383;c3 = ([120 150 230]+128)/383;patch([0 1 1 0],[0 0 1 1],c1);patch([0 1 1 1-e 1-e 0+e],[0 0 1 1-e 0+e 0+e],c2);patch([0 0 1 1-e 0+e 0+e],[0 1 1 1-e 1-e 0+e],c3);plot([0 1 1 0 0],[0 0 1 1 0]);disp('Weights');
  Mux : Mux  Inputs=40
      mask Display: e = 0.06;c1 = [120 150 230]/255;c2 = ([120 150 230]+0)/383;c3 = ([120 150 230]+128)/383;patch([0 1 1 0],[0 0 1 1],c1);patch([0 1 1 1-e 1-e 0+e],[0 0 1 1-e 0+e 0+e],c2);patch([0 0 1 1-e 0+e 0+e],[0 1 1 1-e 1-e 0+e],c3);plot([0 1 1 0 0],[0 0 1 1 0]);disp('Mux');
  dotprod{1..40} (40 alike) : neural/Weight Functions/dotprod
  "iz{1,1}" : Outport
      mask Display: e = 0.06;c1 = [120 230 180]/255;c2 = ([120 230 180]+0)/(256+128);c3 = ([120 230 180]+128)/(256+128);patch([0 1 1 0],[0 0 1 1],c1);patch([0 1 1 1-e 1-e 0+e],[0 0 1 1-e 0+e 0+e],c2);patch([0 0 1 1-e 0+e 0+e],[0 1 1 1-e 1-e 0+e],c3);plot([0 1 1 0 0],[0 0 1 1 0]);
  wires:
  "IW{1,1}(1,:)'"/1 -> dotprod1/1
  "pd{1,1}"/1 -> dotprod1/2, dotprod2/2, dotprod3/2, dotprod4/2, dotprod5/2, dotprod6/2, dotprod7/2, dotprod8/2, dotprod9/2, dotprod10/2, dotprod11/2, dotprod12/2, dotprod13/2, dotprod14/2, dotprod15/2, dotprod16/2, dotprod17/2, dotprod18/2, dotprod19/2, dotprod20/2, dotprod21/2, dotprod22/2, dotprod23/2, dotprod24/2, dotprod25/2, dotprod26/2, dotprod27/2, dotprod28/2, dotprod29/2, dotprod30/2, dotprod31/2, dotprod32/2, dotprod33/2, dotprod34/2, dotprod35/2, dotprod36/2, dotprod37/2, dotprod38/2, dotprod39/2, dotprod40/2
  dotprod1/1 -> Mux/1
  "IW{1,1}(2,:)'"/1 -> dotprod2/1
  dotprod2/1 -> Mux/2
  "IW{1,1}(3,:)'"/1 -> dotprod3/1
  dotprod3/1 -> Mux/3
  "IW{1,1}(4,:)'"/1 -> dotprod4/1
  dotprod4/1 -> Mux/4
  "IW{1,1}(5,:)'"/1 -> dotprod5/1
  dotprod5/1 -> Mux/5
  "IW{1,1}(6,:)'"/1 -> dotprod6/1
  dotprod6/1 -> Mux/6
  "IW{1,1}(7,:)'"/1 -> dotprod7/1
  dotprod7/1 -> Mux/7
  "IW{1,1}(8,:)'"/1 -> dotprod8/1
  dotprod8/1 -> Mux/8
  "IW{1,1}(9,:)'"/1 -> dotprod9/1
  dotprod9/1 -> Mux/9
  "IW{1,1}(10,:)'"/1 -> dotprod10/1
  dotprod10/1 -> Mux/10
  "IW{1,1}(11,:)'"/1 -> dotprod11/1
  dotprod11/1 -> Mux/11
  "IW{1,1}(12,:)'"/1 -> dotprod12/1
  dotprod12/1 -> Mux/12
  "IW{1,1}(13,:)'"/1 -> dotprod13/1
  dotprod13/1 -> Mux/13
  "IW{1,1}(14,:)'"/1 -> dotprod14/1
  dotprod14/1 -> Mux/14
  "IW{1,1}(15,:)'"/1 -> dotprod15/1
  dotprod15/1 -> Mux/15
  "IW{1,1}(16,:)'"/1 -> dotprod16/1
  dotprod16/1 -> Mux/16
  "IW{1,1}(17,:)'"/1 -> dotprod17/1
  dotprod17/1 -> Mux/17
  "IW{1,1}(18,:)'"/1 -> dotprod18/1
  dotprod18/1 -> Mux/18
  "IW{1,1}(19,:)'"/1 -> dotprod19/1
  dotprod19/1 -> Mux/19
  "IW{1,1}(20,:)'"/1 -> dotprod20/1
  dotprod20/1 -> Mux/20
  "IW{1,1}(21,:)'"/1 -> dotprod21/1
  dotprod21/1 -> Mux/21
  "IW{1,1}(22,:)'"/1 -> dotprod22/1
  dotprod22/1 -> Mux/22
  "IW{1,1}(23,:)'"/1 -> dotprod23/1
  dotprod23/1 -> Mux/23
  "IW{1,1}(24,:)'"/1 -> dotprod24/1
  dotprod24/1 -> Mux/24
  "IW{1,1}(25,:)'"/1 -> dotprod25/1
  dotprod25/1 -> Mux/25
  "IW{1,1}(26,:)'"/1 -> dotprod26/1
  dotprod26/1 -> Mux/26
  "IW{1,1}(27,:)'"/1 -> dotprod27/1
  dotprod27/1 -> Mux/27
  "IW{1,1}(28,:)'"/1 -> dotprod28/1
  dotprod28/1 -> Mux/28
  "IW{1,1}(29,:)'"/1 -> dotprod29/1
  dotprod29/1 -> Mux/29
  "IW{1,1}(30,:)'"/1 -> dotprod30/1
  dotprod30/1 -> Mux/30
  "IW{1,1}(31,:)'"/1 -> dotprod31/1
  dotprod31/1 -> Mux/31
  "IW{1,1}(32,:)'"/1 -> dotprod32/1
  dotprod32/1 -> Mux/32
  "IW{1,1}(33,:)'"/1 -> dotprod33/1
  dotprod33/1 -> Mux/33
  "IW{1,1}(34,:)'"/1 -> dotprod34/1
  dotprod34/1 -> Mux/34
  "IW{1,1}(35,:)'"/1 -> dotprod35/1
  dotprod35/1 -> Mux/35
  "IW{1,1}(36,:)'"/1 -> dotprod36/1
  dotprod36/1 -> Mux/36
  "IW{1,1}(37,:)'"/1 -> dotprod37/1
  dotprod37/1 -> Mux/37
  "IW{1,1}(38,:)'"/1 -> dotprod38/1
  dotprod38/1 -> Mux/38
  "IW{1,1}(39,:)'"/1 -> dotprod39/1
  dotprod39/1 -> Mux/39
  "IW{1,1}(40,:)'"/1 -> dotprod40/1
  dotprod40/1 -> Mux/40
  Mux/1 -> "iz{1,1}"/1

== system mrefrobotarm_modified_previous_y_previous_u_previous_ref_Thao/trimmed_cex/Layer 2/Delays 1 ==
  "p{2}" : Inport  PortDimensions=40
      mask Display: e = 0.06;c1 = [120 230 180]/255;c2 = ([120 230 180]+0)/(256+128);c3 = ([120 230 180]+128)/(256+128);patch([0 1 1 0],[0 0 1 1],c1);patch([0 1 1 1-e 1-e 0+e],[0 0 1 1-e 0+e 0+e],c2);patch([0 0 1 1-e 0+e 0+e],[0 1 1 1-e 1-e 0+e],c3);plot([0 1 1 0 0],[0 0 1 1 0]);
  mux : Mux  Inputs=1
      mask Display: e = 0.06;c1 = [120 150 230]/255;c2 = ([120 150 230]+0)/383;c3 = ([120 150 230]+128)/383;patch([0 1 1 0],[0 0 1 1],c1);patch([0 1 1 1-e 1-e 0+e],[0 0 1 1-e 0+e 0+e],c2);patch([0 0 1 1-e 0+e 0+e],[0 1 1 1-e 1-e 0+e],c3);plot([0 1 1 0 0],[0 0 1 1 0]);disp('Mux')
  "pd{2,1}" : Outport
      mask Display: e = 0.06;c1 = [120 230 180]/255;c2 = ([120 230 180]+0)/(256+128);c3 = ([120 230 180]+128)/(256+128);patch([0 1 1 0],[0 0 1 1],c1);patch([0 1 1 1-e 1-e 0+e],[0 0 1 1-e 0+e 0+e],c2);patch([0 0 1 1-e 0+e 0+e],[0 1 1 1-e 1-e 0+e],c3);plot([0 1 1 0 0],[0 0 1 1 0]);
  wires:
  "p{2}"/1 -> mux/1
  mux/1 -> "pd{2,1}"/1
